simulink model "Chotu_undir_hardware"  (R2020a)
settings: Solver=ode15s  StartTime=0.0  StopTime=500  FixedStep=0.01  MaxStep=1e-2  RelTol=1e-4  AbsTol=1e-5
model workspace: external: MAT-File (data not in the file)
undefined symbols (not defined in the file or in its folder): motorIP, motorSP
libraries: arduinosensorlib x5, simulink_extras x1, mobileRoboticsTrainingLib x1
settings Model: Creator=ADMIN  LastModifiedBy=RAJENDRA PHUTANE
settings SolverCC: AutoScaleAbsTol=off
settings ExplorerConfigSet: InternalSimMechanicsExplorerSettings="<ExplorerConfiguration><canonicalview>default</canonicalview><AnimationSetting><BasePlaybackSpeed>1.0</BasePlaybackSpeed><PlaybackSpeedFactor>1.0</PlaybackSpeedFactor></AnimationSetting><TilePanel><TileInfo><Tiles Columns=\"1\" Count=\"1\" Rows=\"1\"><Column Weight=\"1\"/><Row Weight=\"1\"/><Tile Height=\"1\" Width=\"1\" X=\"0\" Y=\"0\"/></Tiles></TileInfo><SceneInfo><SceneViewer><BGColor><R>0.400000005960464478</R><G>0.60000002384185791</G><B>1</B></BGColor><Camera><DoPerspective>on</DoPerspective><Position><X>-0.420479361362930182</X><Y>0.345763219668583144</Y><Z>2.4083672876232054</Z></Position><Center><X>-0.420479361362930182</X><Y>1.31168904595765135</Y><Z>2.14954824252068466</Z></Center><Up><X>0</X><Y>0.258819045102520795</Y><Z>0.965925826289068312</Z></Up><ViewLimDist>1</ViewLimDist><YLim>0.466307658154998583</YLim><XLim>0.802939872047792491</XLim></Camera></SceneViewer></SceneInfo></TilePanel><MechEditorPanel><Cameras><Camera><Id>Camera1</Id><Value><Name>Robot View</Name><NativeCamera><PositionTrackingFeature>Plant_Model.Robot_Camera.F</PositionTrackingFeature><CenterTrackingFeature>Plant_Model.Robot_Camera.F</CenterTrackingFeature><UpVectorTrackingFeature>Plant_Model.Robot_Camera.F</UpVectorTrackingFeature><CenterTrackingOrigin>off</CenterTrackingOrigin><CenterTrackingDirection>+Y</CenterTrackingDirection><UpVectorTrackingDirection>+Z</UpVectorTrackingDirection></NativeCamera></Value></Camera></Cameras><GfxPanelCameraMap><MapElement CameraMLId=\"Camera1\" GfxPanelIndex=\"0\"/></GfxPanelCameraMap><VideoCreator><PlaybackSpeedRatio>1.0</PlaybackSpeedRatio><FrameRate>30</FrameRate><VideoFormat>Motion JPEG AVI</VideoFormat><FrameSize>auto</FrameSize></VideoCreator></MechEditorPanel></ExplorerConfiguration>"

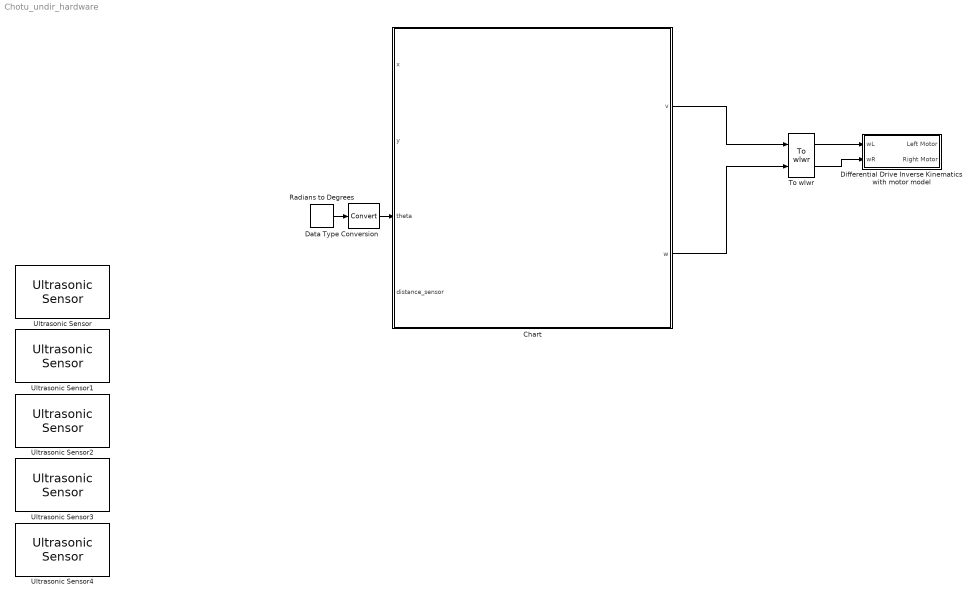
== system Chotu_undir_hardware ==
  Chart : Stateflow chart  TreatAsAtomicUnit=on
  Data Type Conversion : DataTypeConversion
  Differential Drive Inverse Kinematics with motor model : Subsystem
  Radians to Degrees : simulink_extras/Transformations/Radians to Degrees
  To wlwr : mobileRoboticsTrainingLib/To wlwr  axleLength=axleLength  wheelR=wheelR
  Ultrasonic Sensor{,1..4} (5 alike) : arduinosensorlib/Ultrasonic Sensor  NumSignalPins=1  TrigPin=4  EchoPin=5  SignalPin=3  SampleTime_=0.1  blockPlatform=ARDUINO
      settings: SourceProductBaseCode=ARDUINO
  wires:
  Data Type Conversion/1 -> Chart/3(theta)
  Radians to Degrees/1 -> Data Type Conversion/1
  To wlwr/2 -> Differential Drive Inverse Kinematics with motor model/2(wR)
  Chart/1(v) -> To wlwr/1
  To wlwr/1 -> Differential Drive Inverse Kinematics with motor model/1(wL)
  Chart/2(w) -> To wlwr/2

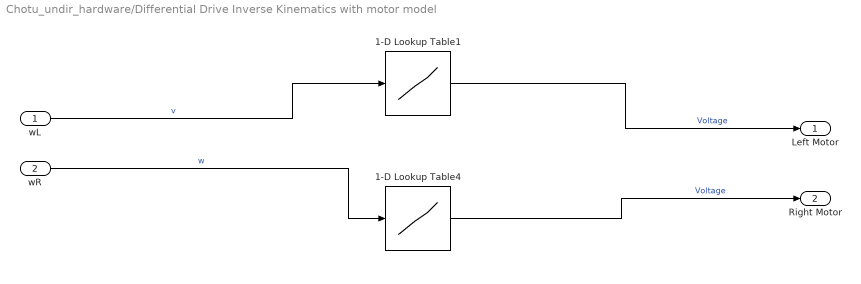
== system Chotu_undir_hardware/Differential Drive Inverse Kinematics with motor model ==
  wL : Inport
  wR : Inport  Port=2
  1-D Lookup Table1 : Lookup_n-D  NumberOfTableDimensions=1  BreakpointsForDimension1=motorSP  Table=motorIP  ExtrapMethod=Clip  InternalRulePriority=Speed  RndMeth=Simplest  InputSameDT=on
  1-D Lookup Table4 : Lookup_n-D  NumberOfTableDimensions=1  BreakpointsForDimension1=motorSP  Table=motorIP  ExtrapMethod=Clip  InternalRulePriority=Speed  RndMeth=Simplest  InputSameDT=on
  Left Motor : Outport  VectorParamsAs1DForOutWhenUnconnected=off
  Right Motor : Outport  Port=2  VectorParamsAs1DForOutWhenUnconnected=off
  wires:
  wL/1 -> 1-D Lookup Table1/1  "v"
  wR/1 -> 1-D Lookup Table4/1  "w"
  1-D Lookup Table4/1 -> Right Motor/1  "Voltage"
  1-D Lookup Table1/1 -> Left Motor/1  "Voltage"

== stateflow chart Chotu_undir_hardware/Chart ==
  state GOSTRAIGHT
    entry:
    dest_theta=0;
    during:
    v=0.5;
    w= 0;
    exit :
    v =0;
    w = 0;
  state TurnLEFT
    entry:
    dest_theta=theta;
    during:
    v = 0.5;
    w = -2;
    exit:
    v =0;
    w = 0;
  state TurnRIGHT
    entry:
    dest_theta=theta;
    during:
    v = 0.5;
    w = 2;
    exit:
    v =0;
    w = 0;
  state TurnRANDOMblockfront
    a=rand;
  state TurnBACKWARD
    entry:
    dest_theta=theta;
    during:
    v=2;
    w=-2;
    exit:
    v=0;
    w=0;
  (default) -> GOSTRAIGHT
  TurnRIGHT -> GOSTRAIGHT : [abs(theta-dest_theta)>= 84]
  TurnLEFT -> GOSTRAIGHT : [abs(theta-dest_theta)>= 84]
  GOSTRAIGHT -> TurnRIGHT [order 1] : [distance_sensor(5)>0.055 &&...
      |  distance_sensor(3)<0.014 &&...
      | distance_sensor(1)<0.055]
  GOSTRAIGHT -> TurnLEFT [order 4] : [distance_sensor(1)>0.055 &&...
      |  distance_sensor(3)<0.014 &&...
      | distance_sensor(5)<0.055]
  GOSTRAIGHT -> TurnBACKWARD [order 3] : [distance_sensor(1)<0.055 &&...
      |  distance_sensor(3)<0.014 &&...
      | distance_sensor(5)<0.055]
  TurnBACKWARD -> GOSTRAIGHT : [abs(theta-dest_theta)>= 174]
  GOSTRAIGHT -> TurnRANDOMblockfront [order 2] : [distance_sensor(1)>0.165 &&...
      |  distance_sensor(3)<0.014 &&...
      | distance_sensor(5)>0.165]
  TurnRANDOMblockfront -> TurnLEFT [order 1] : [a<0.5]
  TurnRANDOMblockfront -> TurnRIGHT [order 2] : [a>=0.5]
  data: x input; y input; theta input; distance_sensor input; dest_theta local; a local; v output; w output
